simulink model "MyPiero_Final"  (R2022b)
settings: Solver=FixedStepDiscrete  StartTime=0.0  StopTime=inf  RelTol=1e-3  EnableMultiTasking=on
model workspace (MAT data in the model file):
  d = 0.18
libraries: arduinolib x4, robotalgslib x1
settings Model: ExtModeTrigDuration=2  Creator=Usuario  LastModifiedBy=Usuario
settings OptimizationCC: ReuseModelBlockBuffer=on  EnhancedBackFolding=on  PassReuseOutputArgsAs=Individual arguments  ZeroExternalMemoryAtStartup=off  ZeroInternalMemoryAtStartup=off  MaxStackSize=64  OptimizeBlockOrder=speed  DifferentSizesBufferReuse=on  EfficientTunableParamExpr=on
settings DebuggingCC: ParameterTunabilityLossMsg=error
settings HardwareCC: ProdBitPerInt=16  ProdBitPerPointer=16  ProdBitPerSizeT=16  ProdBitPerPtrDiffT=16  ProdLargestAtomicFloat=None  ProdWordSize=8  ProdHWDeviceType=Atmel->AVR  UseEmbeddedCoderFeatures=off  UseSimulinkCoderFeatures=off
settings SFSimCC: MATLABDynamicMemAlloc=off
settings RTWCC: Description=Embedded Coder  SystemTargetFile=ert.tlc  HardwareBoard=Arduino Mega 2560  TLCOptions=-aInlineSetEventsForThisBaseRateFcn=TLC_FALSE -aSuppressMultiTaskScheduler=TLC_FALSE -aRateBasedStepFcn=1  TemplateMakefile=ert_default_tmf  Toolchain=Arduino AVR  BuildConfiguration=Faster Runs  GPUComputeCapability=5.0
settings CodeAppCC: ForceParamTrailComments=on  IgnoreCustomStorageClasses=off  OperatorAnnotations=on  SimulinkDataObjDesc=on  SFDataObjDesc=on  InsertBlockDesc=on
settings ERTTargetCC: SupportContinuousTime=on  SupportNonInlinedSFcns=on  SupportVariableSizeSignals=on  ExtModeTransport=3  ExtModeStaticAlloc=on  ExtModeAutomaticAllocSize=off  ExtModeStaticAllocSize=2048  ExtModeMexFile=ext_xcp  ExtModeIntrfLevel=Level2 - Open

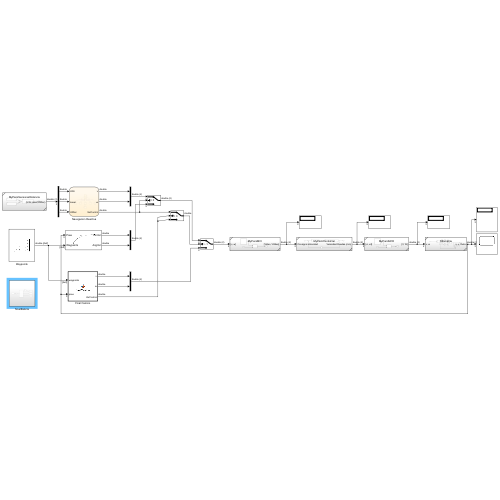
[thumbnail: Simulink's stored preview of the top-level diagram]
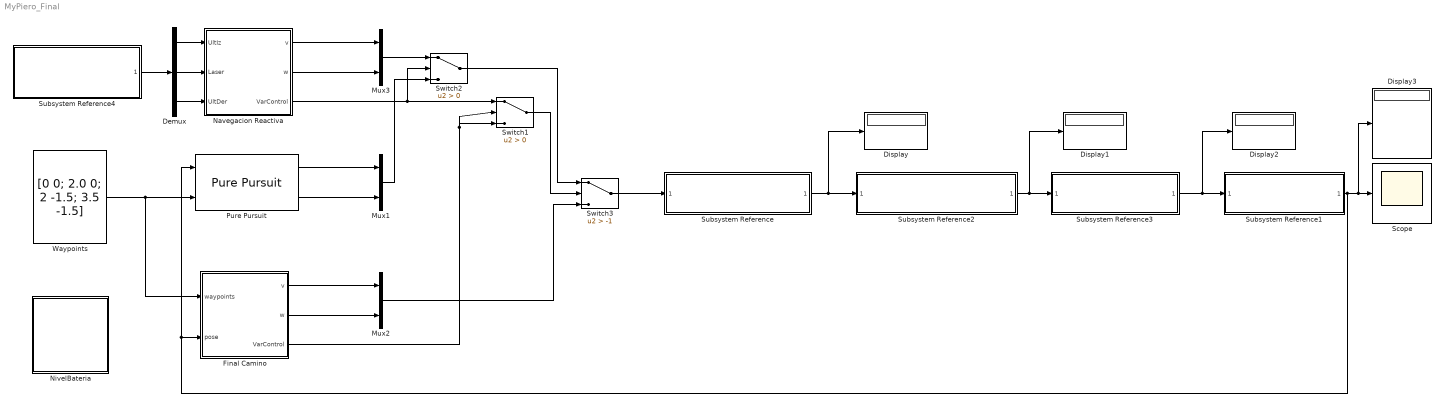
== system MyPiero_Final ==
  Demux : Demux  Outputs=3
  Display{,1..3} (4 alike) : Display
  Final Camino : MATLAB Function  TreatAsAtomicUnit=on
  Mux1 : Mux  Inputs=2
  Mux2 : Mux  Inputs=2
  Mux3 : Mux  Inputs=2
  Navegacion Reactiva : Stateflow chart  TreatAsAtomicUnit=on
  NivelBateria : Subsystem
  Pure Pursuit : robotalgslib/Pure Pursuit  DesiredLinearVelocity=0.3  MaxAngularVelocity=1.5  LookaheadDistance=0.25  TargetDirPort=off  SimulateUsing=Code generation
      settings: LibrarySourceBlock=navlib/Control Algorithms/Pure Pursuit
  Scope : Scope
  Subsystem Reference : Subsystem  ReferencedSubsystem=MyPieroMCI
  Subsystem Reference1 : Subsystem  ReferencedSubsystem=Odometria
  Subsystem Reference2 : Subsystem  ReferencedSubsystem=MyPieroControlVel
  Subsystem Reference3 : Subsystem  ReferencedSubsystem=MyPieroMCD
  Subsystem Reference4 : Subsystem  ReferencedSubsystem=MyPieroSensoresDistancia
  Switch1 : Switch  Criteria=u2 > Threshold  SaturateOnIntegerOverflow=off  InputSameDT=off
  Switch2 : Switch  Criteria=u2 > Threshold  SaturateOnIntegerOverflow=off  InputSameDT=off
  Switch3 : Switch  Criteria=u2 > Threshold  Threshold=-1  SaturateOnIntegerOverflow=off  InputSameDT=off
  Waypoints : Constant  Value=[0 0; 2.0 0; 2 -1.5; 3.5 -1.5]
  wires:
  Subsystem Reference3/1 -> Display2/1, Subsystem Reference1/1
  Subsystem Reference2/1 -> Display1/1, Subsystem Reference3/1
  Subsystem Reference/1 -> Display/1, Subsystem Reference2/1
  Subsystem Reference4/1 -> Demux/1
  Demux/1 -> Navegacion Reactiva/1(UltIz)
  Demux/2 -> Navegacion Reactiva/2(Laser)
  Demux/3 -> Navegacion Reactiva/3(UltDer)
  Waypoints/1 -> Final Camino/1(waypoints), Pure Pursuit/2
  Subsystem Reference1/1 -> Display3/1, Scope/1, Pure Pursuit/1, Final Camino/2(pose)
  Final Camino/1(v) -> Mux2/1
  Final Camino/2(w) -> Mux2/2
  Navegacion Reactiva/2(w) -> Mux3/2
  Navegacion Reactiva/1(v) -> Mux3/1
  Mux2/1 -> Switch3/3
  Switch3/1 -> Subsystem Reference/1
  Navegacion Reactiva/3(VarControl) -> Switch2/2, Switch1/1
  Final Camino/3(VarControl) -> Switch1/3, Switch1/2
  Switch1/1 -> Switch3/2
  Switch2/1 -> Switch3/1
  Mux3/1 -> Switch2/1
  Mux1/1 -> Switch2/3
  Pure Pursuit/2 -> Mux1/2
  Pure Pursuit/1 -> Mux1/1

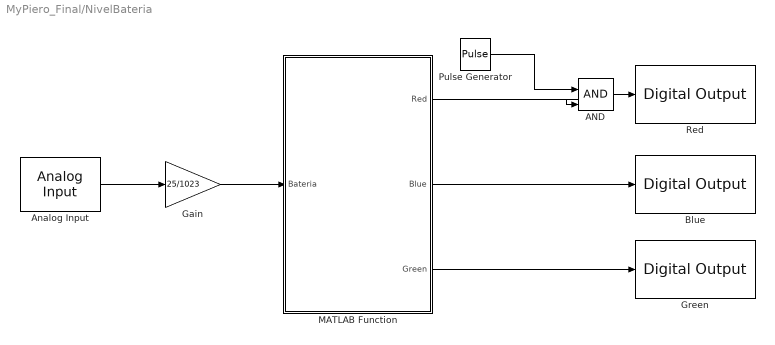
== system MyPiero_Final/NivelBateria ==
  AND : Logic  IconShape=distinctive  AllPortsSameDT=off  OutDataTypeStr=boolean
  Analog Input : arduinolib/Analog Input  pinNumber=0  ReadResultsOnly=off  ConversionTriggerSource=Software  ExternalTriggerType=uint32( 0 )  OutputDataType=uint16  EnableConversionCompleteNotify=off  EnableOuputStatus=off  SampleTime=-1  blockPlatform=arduino
  Blue : arduinolib/Digital Output  pinNumber=13  Direction=output  blockPlatform=arduino
  Gain : Gain  Gain=25/1023
  Green : arduinolib/Digital Output  pinNumber=11  Direction=output  blockPlatform=arduino
  MATLAB Function : MATLAB Function  TreatAsAtomicUnit=on
  Pulse Generator : DiscretePulseGenerator  PulseType=Time based  Period=1  PulseWidth=5
  Red : arduinolib/Digital Output  pinNumber=12  Direction=output  blockPlatform=arduino
  wires:
  AND/1 -> Red/1
  Gain/1 -> MATLAB Function/1(Bateria)
  MATLAB Function/2(Blue) -> Blue/1
  Pulse Generator/1 -> AND/1
  MATLAB Function/1(Red) -> AND/2
  Analog Input/1 -> Gain/1
  MATLAB Function/3(Green) -> Green/1

== matlab function MyPiero_Final/NivelBateria/MATLAB Function ==
  data: Bateria input; Red output; Blue output; Green output
function [Red,Blue,Green] = NivelBateria(Bateria)
if (Bateria >= 12.1)
    Green = 1;
    Blue = 0;
    Red = 0;
elseif ((Bateria < 12.1) &&(Bateria >= 11.5))
    Green = 0;
    Blue = 1;
    Red = 0;
else
    Green = 0;
    Blue = 0;
    Red = 1;
end

== stateflow chart MyPiero_Final/Navegacion Reactiva ==
  state TightWay
    % Con esto intentare que
    % pase por un camino
    % estrecho hasta donde
    % pueda
    entry:
    VarControl = 1;
    v = 0.5;
    w = 0;
  state FullRotation
    % Si detecta algo
    % en todos los sentidos
    entry:
    VarControl = 1;
    v = 0;
    w = -pi + 0.1;
  state Default
    entry:
    VarControl = 0;
    v = 0.2;
    w = 0;
  state LeftSonar_Far
    % Si solo detecta el
    % Obstaculo con el
    % ultrasonidos izquierdo
    % lejos
    entry:
    VarControl = 1;
    v = 0.2;
    w = -pi/8;
  state LeftSonar_Close
    % Si solo detecta el
    % Obstaculo con el
    % ultrasonidos izquierdo
    % cerca
    entry:
    VarControl = 1;
    v = 0;
    w = -pi/4;
  state MidLaser
    entry:
    VarControl = 1;
    v = 0;
    w = 0;
    % Calculo el signo para
    % la rotacion aleatoria
    if round(rand) == 0
    sign = -1;
    else
    sign = 1;
    end
  state RightSonar_Close
    % Si solo detecta el
    % Obstaculo con el
    % ultrasonidos derecho
    % cerca
    entry:
    VarControl = 1;
    v = 0;
    w = pi/4;
  state RightSonar_Far
    % Si solo detecta el
    % Obstaculo con el
    % ultrasonidos izquierdo
    % lejos
    entry:
    VarControl = 1;
    v = 0.2;
    w = pi/8;
  state RandomRotation
    % Si solo detecta el
    % Obstaculo con el
    % Laser
    entry:
    VarControl = 1;
    v =  0;
    w = sign*pi/4;
  TightWay -> TightWay [order 2] : [(UltIz > 12) && (UltDer >12)]
  Default -> TightWay [order 2] : [(UltIz < 25) && (Laser >= 20) && (UltDer < 25)]
  TightWay -> FullRotation [order 3] : [(UltIz <= 12) && (UltDer <= 12)]
  TightWay -> Default [order 1] : after(0.1,sec)
  FullRotation -> FullRotation [order 1] : [Laser < 25]
  Default -> FullRotation [order 1] : [(UltIz < 25) && (Laser < 20) && (UltDer < 25)]
  FullRotation -> Default [order 2] : after(0.1, sec)
  (default) -> Default
  Default -> RightSonar_Far [order 5] : [(UltDer < 30) && (UltDer >= 20)]
  Default -> LeftSonar_Far [order 4] : [(UltIz < 30) && (UltIz >= 20)]
  RightSonar_Far -> Default [order 1] : [(UltDer >= 30) || (UltDer < 20)]
  LeftSonar_Far -> Default [order 1] : [(UltIz >= 30) || (UltIz < 20)]
  RightSonar_Close -> Default [order 1] : [UltDer >= 20]
  LeftSonar_Close -> Default [order 1] : [UltIz >= 20 ]
  Default -> RightSonar_Close [order 7] : [UltDer < 20]
  Default -> LeftSonar_Close [order 6] : [UltIz < 20]
  Default -> MidLaser [order 3] : [Laser < 20]
  MidLaser -> Default [order 1] : [Laser > 25]
  LeftSonar_Far -> LeftSonar_Far [order 2] : [(UltIz < 30) && (UltIz >= 20)]
  RightSonar_Far -> RightSonar_Far [order 2] : [(UltDer < 30) && (UltDer >= 20)]
  LeftSonar_Close -> LeftSonar_Close [order 2] : [UltIz < 20]
  RightSonar_Close -> RightSonar_Close [order 2] : [UltDer < 20]
  MidLaser -> RandomRotation [order 2] : after(0.1,sec)
  RandomRotation -> MidLaser [order 1] : after(0.2,sec)
  RandomRotation -> RandomRotation [order 2] : [Laser <= 25]
  data: UltIz input; Laser input; UltDer input; v output; w output; sign local; VarControl output

== matlab function MyPiero_Final/Final Camino ==
  data: waypoints input; v output double size=1; pose input; w output double size=1; VarControl output size=1
function [v,w,VarControl] = FinalCamino(waypoints, pose)
PoseX = pose(1); 
PoseY = pose(2);

w = 0;

[N,~] = size(waypoints);
XFin = waypoints(N,1);
YFin = waypoints(N,2);

if ((PoseX <= (XFin + 0.2)) && (PoseX >= (XFin - 0.2))) && ((PoseY <= (YFin + 0.2)) && (PoseY >= (YFin - 0.2)))  
    VarControl = -1;
    v = 0;
else
    VarControl = 0;
    v = 0.3;
end
